simulink library "Radiator"  (R2018b)
settings: Solver=ode45  StartTime=0.0  StopTime=10.0  RelTol=1e-3  EnableMultiTasking=on
libraries: carnot x2
settings Model: Creator=lena.frank  LastModifiedBy=drhf
settings DataIOCC: LimitDataPoints=on  SaveFormat=Array  SignalLoggingSaveFormat=ModelDataLogs
settings OptimizationCC: ExpressionDepthLimit=2147483647  LifeSpan=inf
settings DebuggingCC: UnderspecifiedInitializationDetection=Classic  MergeDetectMultiDrivingBlocksExec=none  SolverPrmCheckMsg=warning  FcnCallInpInsideContextMsg=warning  StateNameClashWarn=warning  SFUnexpectedBacktrackingDiag=warning  SFNoUnconditionalDefaultTransitionDiag=warning  SFExecutionAtInitializationDiag=none
settings HardwareCC: ProdBitPerPointer=32  ProdBitPerSizeT=32  ProdBitPerPtrDiffT=32  ProdLargestAtomicFloat=None  ProdIntDivRoundTo=Undefined  ProdEndianess=Unspecified  ProdWordSize=32  ProdHWDeviceType=32-bit Generic
settings ModelReferenceCC: PropagateSignalLabelsOutOfModel=off
settings SFSimCC: SimUseLocalCustomCode=off
settings RTWCC: RTWUseLocalCustomCode=off
settings CodeAppCC: StateflowObjectComments=on
settings GRTTargetCC: TargetLangStandard=C89/C90 (ANSI)  GeneratePreprocessorConditionals=Disable all  CombineOutputUpdateFcns=off  GRTInterface=on
settings ConfigComp: CovMetricSettings=dw  CovHtmlReporting=on  CovSaveCumulativeToWorkspaceVar=on  CovSaveSingleToWorkspaceVar=on  CovExternalEMLEnable=off

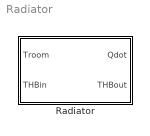
== system Radiator ==
  Radiator : Subsystem  mask(Radiator){pnom=500, dtnom=49.83, expo=1.3, mcap=5*4182, tini=20, lin=10, qua=10}
      mask prompts: pnom "Qdot_nom: nominal power in W"; dtnom "Tdiff_nom: nominal temperature difference in K"; expo "radiator exponent (> 0)"; mcap "mass * capacity per unit in J/K"; tini "Initial temperature in °C"; lin "l : linear pressure drop Pa/(kg/s)"; qua "q : quadratic pressure drop Pa/(kg/s)²"
      mask help:
      | Calculates the power of a radiator according to the nominal power the and the temperature difference (EN 442).
      | Qdot = Qdot_nom * (Tdiff/Tdiff_nom)^exponent
      | Tdiff_nom for EN 442 test is 49.83 K
      | The thermal capacity of the radiator is modeled by a 1-node capacity.
      | mcp*dTnode/dt = mdot*cp*(Tin-Tnode)-Qdot
      | In difference to EN 442 the outlet temperature is Tnode. Tnode is not calculated as average temperature of inlet and outlet.
      | A quadratic pressure drop is applied to the fluid flow.
      mask Help: web(['file:///' fullfile(path_carnot('help'),'Radiator.html')],'-helpbrowser')
      mask TypeOptions pnom: Radiator_basic/pnomEN
      mask TypeOptions dtnom: Radiator_basic/dtnomEN
      mask TypeOptions expo: Radiator_basic/expo
      mask TypeOptions mcap: Radiator_basic/mcp
      mask TypeOptions tini: Radiator_basic/tini
      mask TypeOptions lin: pressdrop_fix_THB/lin
      mask TypeOptions qua: pressdrop_fix_THB/qua
      mask DialogControl ParameterTabVar0 Prompt: Thermal
      mask DialogControl ParameterTabVar01 Prompt: Hydraulic
      mask Display: plot(-20,0,120,90,[20 90 90 20 20],[20 20 70 70 20],[30 30],[25 65],[40 40],[25 65],[50 50],[25 65],[60 60],[25 65],[70 70],[25 65],[80 80],[25 65],[15 20],[25 25],[15 20],[65 65])

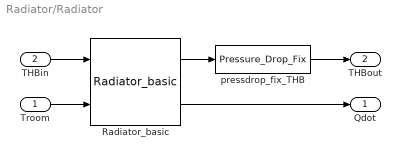
== system Radiator/Radiator ==
  Troom : Inport
  THBin : Inport  Port=2
  Radiator_basic : carnot/Basic/Thermal_Models/Radiator_basic  pnomEN=pnom  dtnomEN=dtnom  expo=expo  mcp=mcap  tini=tini
      settings: SourceProductName=Carnot
  pressdrop_fix_THB : carnot/Basic/Pressure_Drop/Pressure_Drop_Fix  con=0  lin=lin  qua=qua
      settings: SourceProductName=Carnot
  Qdot : Outport
  THBout : Outport  Port=2
  wires:
  Radiator_basic/2 -> Qdot/1
  Troom/1 -> Radiator_basic/2
  THBin/1 -> Radiator_basic/1
  Radiator_basic/1 -> pressdrop_fix_THB/1
  pressdrop_fix_THB/1 -> THBout/1
